simulink model "Modell_PT1_mit_Winkel"  (R2020a)
settings: Solver=VariableStepAuto  StartTime=0.0  StopTime=10.0  RelTol=1e-3
libraries: simulink x2
settings Model: Creator=nicol  LastModifiedBy=nicol

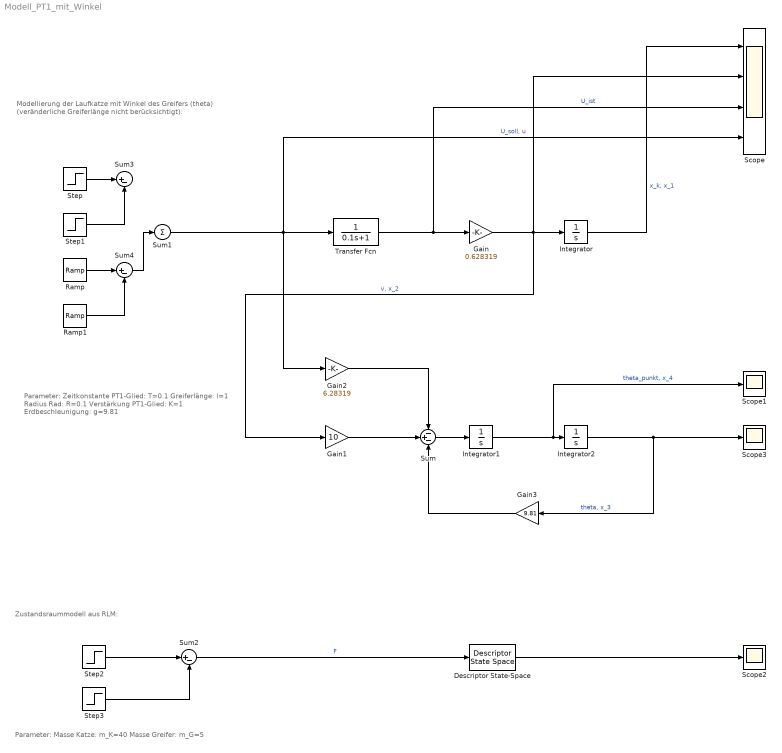
== system Modell_PT1_mit_Winkel ==
  note: Parameter:
      | Masse Katze: m_K=40
      | Masse Greifer: m_G=5
  note: Zustandsraummodell aus RLM:
  note: Modellierung der Laufkatze mit Winkel des Greifers (theta) (veränderliche Greiferlänge nicht berücksichtigt):
  note: Parameter:
      | Zeitkonstante PT1-Glied: T=0.1
      | Greiferlänge: l=1
      | Radius Rad: R=0.1
      | Verstärkung PT1-Glied: K=1
      | Erdbeschleunigung: g=9.81
  Descriptor State-Space : DescriptorStateSpace  E=[1 0 0 0; 0 1 0 0; 0 0 1 0; 0 0 0 1]  A=[0 1 0 0; 0 0 1.226 0; 0 0 0 1; 0 0 -11.036 0]  B=[0; 0.025; 0; -0.025]  C=[1 0 0 0; 0 1 0 0; 0 0 1 0; 0 0 0 1]  D=[0; 0; 0; 0]
  Gain : Gain  Gain=0.628319
  Gain1 : Gain  Gain=10
  Gain2 : Gain  Gain=6.28319
  Gain3 : Gain  Gain=9.81
  Integrator : Integrator
  Integrator1 : Integrator
  Integrator2 : Integrator
  Ramp : simulink/Sources/Ramp  slope=0.1  start=1  InitialOutput=0
  Ramp1 : simulink/Sources/Ramp  slope=0.1  start=5  InitialOutput=0
  Scope : Scope  NumInputPorts=4
  Scope1 : Scope
  Scope2 : Scope
  Scope3 : Scope
  Step : Step  SampleTime=0
  Step1 : Step  Time=4  SampleTime=0
  Step2 : Step  After=10  SampleTime=0
  Step3 : Step  Time=5  After=10  SampleTime=0
  Sum : Sum  Inputs=-+-
  Sum1 : Sum  Inputs=|+|
  Sum2 : Sum  Inputs=|+-
  Sum3 : Sum  Inputs=|+-
  Sum4 : Sum  Inputs=|+-
  Transfer Fcn : TransferFcn  Denominator=[0.1,1]
  wires:
  Transfer Fcn/1 -> Scope/3, Gain/1  "U_ist"
  Gain/1 -> Scope/2, Integrator/1, Gain1/1  "v, x_2"
  Integrator/1 -> Scope/1  "x_k, x_1"
  Gain2/1 -> Sum/1
  Sum/1 -> Integrator1/1
  Integrator1/1 -> Scope1/1, Integrator2/1  "theta_punkt, x_4"
  Integrator2/1 -> Gain3/1, Scope3/1  "theta, x_3"
  Gain3/1 -> Sum/3
  Gain1/1 -> Sum/2
  Sum1/1 -> Scope/4, Transfer Fcn/1, Gain2/1  "U_soll, u"
  Descriptor State-Space/1 -> Scope2/1
  Step3/1 -> Sum2/2
  Step2/1 -> Sum2/1
  Sum2/1 -> Descriptor State-Space/1  "F"
  Step/1 -> Sum3/1
  Step1/1 -> Sum3/2
  Ramp/1 -> Sum4/1
  Ramp1/1 -> Sum4/2
  Sum4/1 -> Sum1/1
